simulink model "sampleModel51"  (R2021b)
settings: Solver=VariableStepAuto  StartTime=0.0  StopTime=10.0  RelTol=1e-3
undefined symbols (not defined in the file or in its folder): DiscIntNeverNeededParam, Newton, Raphson
libraries: simulink x10
settings Model: Creator=user  LastModifiedBy=user

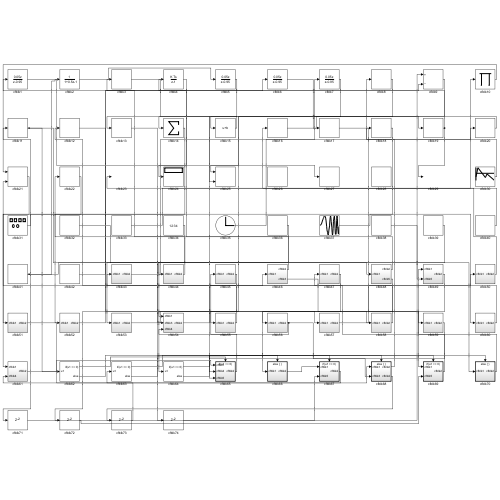
[thumbnail: Simulink's stored preview of the top-level diagram]
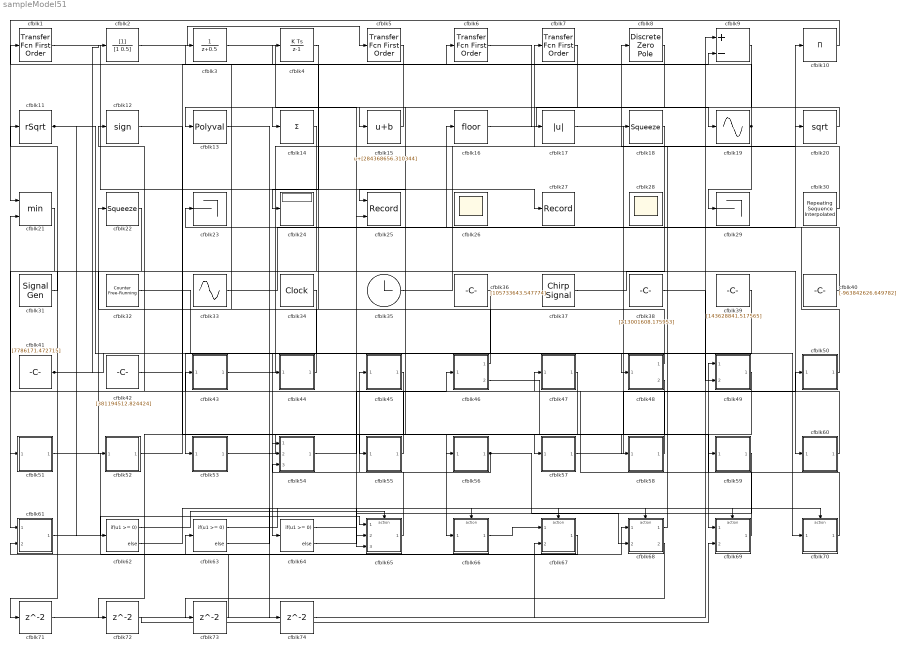
== system sampleModel51 ==
  cfblk{1,5..7} (4 alike) : simulink/Discrete/Transfer Fcn First Order  PoleZ=0.95  ICPrevOutput=0.0  DoSatur=off
  cfblk10 : Product  Inputs=*
  cfblk11 : Sqrt  Operator=rSqrt  AlgorithmType=Newton-Raphson  SaturateOnIntegerOverflow=on
  cfblk12 : Signum
  cfblk13 : Polyval  Coefs=[ +2.081618890e-019, -1.441693666e-014, +4.719686976e-010, -8.536869453e-006, +1.621573104e-001, -8.087801117e+001 ]
  cfblk14 : Sum  Inputs=+
  cfblk15 : Bias  Bias=[284368656.310344]
  cfblk16 : Rounding
  cfblk17 : Abs
  cfblk18 : Squeeze
  cfblk19 : Sin  TimeSource=Use external signal  SampleTime=0
  cfblk2 : DiscreteFilter  SampleTime=1
  cfblk20 : Sqrt  SaturateOnIntegerOverflow=on
  cfblk21 : MinMax  Inputs=2
  cfblk22 : Squeeze
  cfblk23 : Terminator
  cfblk24 : Display
  cfblk25 : Record  FileSettingsInternal="{\"entries\":[{\"content\":{\"excelSettings\":{\"content\":{},\"type\":\"Streamout.ExcelSettings\"}},\"type\":\"Streamout.FileSettingStorage\",\"uuid\":\"25a07257-a86f-477b-952e-0e759ef5e051\"}],\"packageUris\":[\"http://schema.mathworks.com/mf0/streamout_blocks/R2020a\"],\"version\":\"1.0\"}"  Layout=[1 1]  SignalsInternal="{\"entries\":[{\"content\":{\"signals\":[{\"content\":{\"blockPath\":[\"sampleModel51/cfblk25\"],\"channel\":[],\"dimensions\":[1],\"domain\":\"sampleModel51/cfblk25\",\"lineColor\":\"#a2142f\",\"plots\":[1],\"port\":1,\"sid\":[\"\"],\"signalID\":1857,\"signalName\":\"cfblk7\"},\"type\":\"RecordBlkView.Signal\",\"uuid\":\"bc7b99ac-22d1-4a7a-8eb9-f05fbf7987ad\"},{\"content\":{\"blockPath\":[\"sampleModel51/cfblk25\"],\"channel\":[],\"dimensions\":[1],\"domain\":\"sampleModel51/cfblk25\",\"lineColor\":\"#139fff\",\"plots\":[1],\"port\":2,\"sid\":[\"\"],\"signalID\":1861,\"signalName\":\"cfblk8\"},\"type\":\"RecordBlkView.Signal\",\"uuid\":\"eec4487d-860f-4009-9e4b-d7d68678033c\"}]},\"type\":\"RecordBlkView.InputSignals\",\"uuid\":\"330df4c9-4a7c-4ca9-881d-def7613869be\"}],\"packageUris\":[\"http://schema.mathworks.com/mf0/streamout_blocks/R2020a\"],\"version\":\"1.0\"}"  VisualizationBindings="{\"xyplotplugin\":{\"info\":[{\"series\":[{\"bindingParametersList\":[{\"parameter\":\"X-Axis\",\"signalID\":1857,\"signalName\":\"cfblk7\"},{\"parameter\":\"Y-Axis\",\"signalID\":1861,\"signalName\":\"cfblk8\"}],\"seriesID\":23151}],\"subplotID\":1}]}}"  CompatibilityTag=XY
  cfblk26 : Scope
      settings: Floating=on
  cfblk27 : Record  FileSettingsInternal="{\"entries\":[{\"content\":{\"excelSettings\":{\"content\":{},\"type\":\"Streamout.ExcelSettings\"}},\"type\":\"Streamout.FileSettingStorage\",\"uuid\":\"a12ccd90-a1d8-4ecd-8f26-21958fc88e0b\"}],\"packageUris\":[\"http://schema.mathworks.com/mf0/streamout_blocks/R2020a\"],\"version\":\"1.0\"}"  SignalsInternal="{\"entries\":[{\"content\":{\"signals\":[{\"content\":{\"blockPath\":[\"sampleModel51/cfblk27\"],\"channel\":[],\"dimensions\":[1],\"domain\":\"sampleModel51/cfblk27\",\"lineColor\":\"#b746ff\",\"plots\":[1],\"port\":1,\"sid\":[\"\"],\"signalID\":1853,\"signalName\":\"cfblk1\"},\"type\":\"RecordBlkView.Signal\",\"uuid\":\"1f1b1c54-a698-4fa8-9717-1515f275c3ed\"}]},\"type\":\"RecordBlkView.InputSignals\",\"uuid\":\"6aba2456-39ed-4904-9406-7c7f8254458a\"}],\"packageUris\":[\"http://schema.mathworks.com/mf0/streamout_blocks/R2020a\"],\"version\":\"1.0\"}"  VisualizationBindings="{\"sparklinesplugin\":{\"info\":[{\"bindingParametersList\":[],\"subplotID\":1}]}}"
  cfblk28 : Scope
      settings: Floating=on
  cfblk29 : Terminator
  cfblk3 : DiscreteTransferFcn  SampleTime=1
  cfblk30 : simulink/Sources/Repeating Sequence Interpolated  OutValues=[-278627430.459222, 439164858.532469, -328851896.173823, -43963004.255277, -552329955.086711]  TimeValues=[0 0.1 0.5 0.6 1].'  LookUpMeth=Use Input Nearest  tsamp=0.01  OutMin=[]  OutMax=[]  OutDataTypeStr=double  OutputDataTypeScalingMode=double  OutDataType=fixdt(0,8)  OutScaling=2^-10
  cfblk31 : SignalGenerator  Amplitude=[243590977.755836]  Units=rad/sec
  cfblk32 : simulink/Sources/Counter Free-Running  NumBits=[9.000000]  tsamp=-1
  cfblk33 : Sin  Amplitude=[-822452745.496460]  Bias=[355937665.423615]  SampleTime=0
  cfblk34 : DigitalClock
  cfblk35 : Clock
  cfblk36 : Constant  Value=[105733643.547774]  SampleTime=1
  cfblk37 : simulink/Sources/Chirp Signal  f1=[-199962809.726746]  T=[147891668.344843]  f2=[-456672976.291181]
  cfblk38 : Constant  Value=[213001608.175953]  SampleTime=1
  cfblk39 : Constant  Value=[143628841.517565]  SampleTime=1
  cfblk4 : DiscreteIntegrator  ICPrevOutput=DiscIntNeverNeededParam  ICPrevScaledInput=DiscIntNeverNeededParam
  cfblk40 : Constant  Value=[-963842626.649782]  SampleTime=1
  cfblk41 : Constant  Value=[7786171.472715]  SampleTime=1
  cfblk42 : Constant  Value=[381194512.824424]  SampleTime=1
  cfblk43 : Subsystem
  cfblk44 : Subsystem
  cfblk45 : Subsystem
  cfblk46 : Subsystem
  cfblk47 : Subsystem
  cfblk48 : Subsystem
  cfblk49 : Subsystem
  cfblk50 : Subsystem
  cfblk51 : Subsystem
  cfblk52 : Subsystem
  cfblk53 : Subsystem
  cfblk54 : Subsystem
  cfblk55 : Subsystem
  cfblk56 : Subsystem
  cfblk57 : Subsystem
  cfblk58 : Subsystem
  cfblk59 : Subsystem
  cfblk60 : Subsystem
  cfblk61 : Subsystem
  cfblk62 : If  IfExpression=u1 >= 0  SampleTime=1
  cfblk63 : If  IfExpression=u1 >= 0  SampleTime=1
  cfblk64 : If  IfExpression=u1 >= 0  SampleTime=1
  cfblk65 : Subsystem  TreatAsAtomicUnit=on
  cfblk66 : Subsystem  TreatAsAtomicUnit=on
  cfblk67 : Subsystem  TreatAsAtomicUnit=on
  cfblk68 : Subsystem  TreatAsAtomicUnit=on
  cfblk69 : Subsystem  TreatAsAtomicUnit=on
  cfblk70 : Subsystem  TreatAsAtomicUnit=on
  cfblk{71..74} (4 alike) : Delay  SampleTime=1
  cfblk8 : DiscreteZeroPole  Poles=[0 0.5]  Gain=1
  cfblk9 : Sum  Inputs=+-
  wires:
  cfblk65/1(cfblk2) -> cfblk45/1(cfblk1)
  cfblk39/1 -> cfblk53/1(cfblk1)
  cfblk2/1 -> cfblk5/1
  cfblk51/1(cfblk2) -> cfblk68/1(cfblk1)
  cfblk61/1(cfblk2) -> cfblk65/1(cfblk1)
  cfblk37/1 -> cfblk60/1(cfblk1)
  cfblk16/1 -> cfblk19/1
  cfblk1/1 -> cfblk27/1
  cfblk50/1(cfblk2) -> cfblk23/1
  cfblk44/1(cfblk2) -> cfblk22/1
  cfblk69/1(cfblk2) -> cfblk49/1(cfblk1)
  cfblk5/1 -> cfblk14/1
  cfblk59/1(cfblk2) -> cfblk65/2(cfblk4)
  cfblk10/1 -> cfblk21/1
  cfblk57/1(cfblk2) -> cfblk50/1(cfblk1)
  cfblk41/1 -> cfblk2/1, cfblk48/1(cfblk1)
  cfblk15/1 -> cfblk13/1
  cfblk12/1 -> cfblk58/1(cfblk1)
  cfblk35/1 -> cfblk7/1
  cfblk31/1 -> cfblk11/1
  cfblk60/1(cfblk2) -> cfblk12/1
  cfblk40/1 -> cfblk16/1
  cfblk33/1 -> cfblk10/1
  cfblk36/1 -> cfblk64/1
  cfblk47/1(cfblk2) -> cfblk66/1(cfblk1)
  cfblk38/1 -> cfblk49/2(cfblk5)
  cfblk55/1(cfblk2) -> cfblk43/1(cfblk1)
  cfblk9/1 -> cfblk55/1(cfblk1)
  cfblk32/1 -> cfblk70/1(cfblk1)
  cfblk54/1(cfblk2) -> cfblk46/1(cfblk1)
  cfblk49/1(cfblk2) -> cfblk56/1(cfblk1)
  cfblk20/1 -> cfblk15/1
  cfblk58/1(cfblk2) -> cfblk21/2
  cfblk17/1 -> cfblk69/1(cfblk1)
  cfblk30/1 -> cfblk8/1
  cfblk52/1(cfblk2) -> cfblk6/1
  cfblk22/1 -> cfblk61/1(cfblk1)
  cfblk53/1(cfblk2) -> cfblk57/1(cfblk1)
  cfblk6/1 -> cfblk17/1
  cfblk70/1(cfblk2) -> cfblk47/1(cfblk1)
  cfblk3/1 -> cfblk65/3(cfblk5)
  cfblk66/1(cfblk2) -> cfblk67/1(cfblk1)
  cfblk68/1(cfblk2) -> cfblk18/1
  cfblk43/1(cfblk2) -> cfblk20/1
  cfblk21/1 -> cfblk51/1(cfblk1)
  cfblk4/1 -> cfblk24/1
  cfblk46/1(cfblk2) -> cfblk4/1
  cfblk67/1(cfblk2) -> cfblk61/2(cfblk4)
  cfblk7/1 -> cfblk25/1
  cfblk14/1 -> cfblk52/1(cfblk1)
  cfblk42/1 -> cfblk9/2
  cfblk8/1 -> cfblk25/2
  cfblk56/1(cfblk2) -> cfblk68/2(cfblk3), cfblk54/3(cfblk4)
  cfblk11/1 -> cfblk44/1(cfblk1), cfblk62/1
  cfblk46/2(cfblk3) -> cfblk59/1(cfblk1)
  cfblk19/1 -> cfblk29/1, cfblk1/1
  cfblk48/1(cfblk2) -> cfblk3/1
  cfblk48/2(cfblk5) -> cfblk54/1(cfblk1)
  cfblk34/1 -> cfblk54/2(cfblk3)
  cfblk62/1 -> cfblk65/Action
  cfblk62/2 -> cfblk66/Action
  cfblk63/1 -> cfblk67/Action
  cfblk63/2 -> cfblk68/Action
  cfblk64/1 -> cfblk69/Action
  cfblk64/2 -> cfblk70/Action
  cfblk18/1 -> cfblk71/1
  cfblk71/1 -> cfblk67/2(cfblk5)
  cfblk45/1(cfblk2) -> cfblk72/1
  cfblk72/1 -> cfblk69/2(cfblk5)
  cfblk68/2(cfblk4) -> cfblk73/1
  cfblk73/1 -> cfblk63/1
  cfblk13/1 -> cfblk74/1
  cfblk74/1 -> cfblk9/1

== system sampleModel51/cfblk43 ==
  cfblk1 : Inport
  cfblk3 : Product  Inputs=*
  cfblk2 : Outport
  wires:
  cfblk1/1 -> cfblk2/1, cfblk3/1

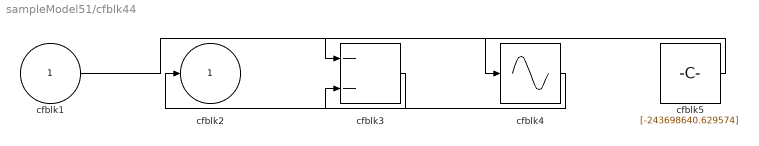
== system sampleModel51/cfblk44 ==
  cfblk1 : Inport
  cfblk3 : Sum  Inputs=--
  cfblk4 : Sin  TimeSource=Use external signal  SampleTime=0
  cfblk5 : Constant  Value=[-243698640.629574]  SampleTime=1
  cfblk2 : Outport
  wires:
  cfblk5/1 -> cfblk3/1
  cfblk3/1 -> cfblk2/1
  cfblk4/1 -> cfblk3/2
  cfblk1/1 -> cfblk4/1

== system sampleModel51/cfblk45 ==
  cfblk1 : Inport
  cfblk3 : Bias  Bias=[345475701.339548]
  cfblk2 : Outport
  wires:
  cfblk1/1 -> cfblk3/1
  cfblk3/1 -> cfblk2/1

== system sampleModel51/cfblk46 ==
  cfblk1 : Inport
  cfblk2 : Outport
  cfblk3 : Outport  Port=2
  wires:
  cfblk1/1 -> cfblk3/1, cfblk2/1

== system sampleModel51/cfblk47 ==
  cfblk1 : Inport
  cfblk3 : Sqrt  SaturateOnIntegerOverflow=on
  cfblk2 : Outport
  wires:
  cfblk1/1 -> cfblk3/1
  cfblk3/1 -> cfblk2/1

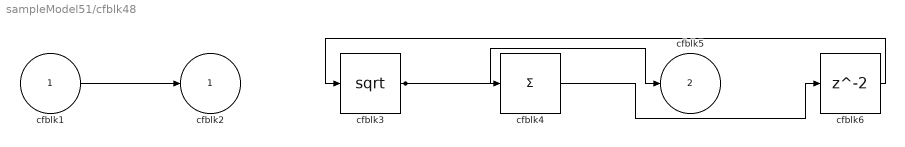
== system sampleModel51/cfblk48 ==
  cfblk1 : Inport
  cfblk3 : Sqrt  SaturateOnIntegerOverflow=on
  cfblk4 : Sum  Inputs=+
  cfblk6 : Delay  SampleTime=1
  cfblk2 : Outport
  cfblk5 : Outport  Port=2
  wires:
  cfblk3/1 -> cfblk5/1, cfblk4/1
  cfblk1/1 -> cfblk2/1
  cfblk4/1 -> cfblk6/1
  cfblk6/1 -> cfblk3/1

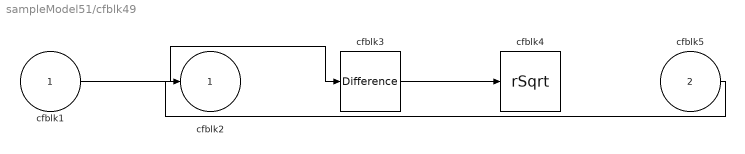
== system sampleModel51/cfblk49 ==
  cfblk1 : Inport
  cfblk5 : Inport  Port=2
  cfblk3 : simulink/Discrete/Difference  ICPrevInput=0.0  OutMin=[]  OutMax=[]  OutDataTypeStr=Inherit: Inherit via back propagation  OutDataType=fixdt(1, 16)  OutScaling=2^-10  DoSatur=off
  cfblk4 : Sqrt  Operator=rSqrt  AlgorithmType=Newton-Raphson  SaturateOnIntegerOverflow=on
  cfblk2 : Outport
  wires:
  cfblk3/1 -> cfblk4/1
  cfblk1/1 -> cfblk3/1
  cfblk5/1 -> cfblk2/1

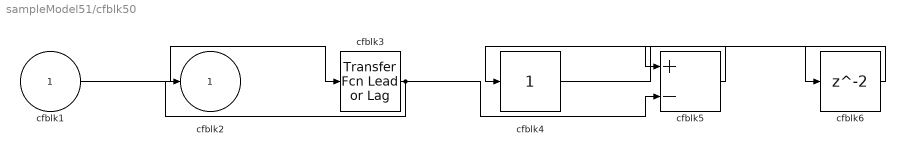
== system sampleModel51/cfblk50 ==
  cfblk1 : Inport
  cfblk3 : simulink/Discrete/Transfer Fcn Lead or Lag  PoleZ=0.95  ZeroZ=0.75  ICPrevOutput=0.0  ICPrevInput=0.0  DoSatur=off
      settings: SourceProductBaseCode=SL
  cfblk4 : simulink/Math Operations/Slider Gain  gain=1  low=0  high=2
  cfblk5 : Sum  Inputs=+-
  cfblk6 : Delay  SampleTime=1
  cfblk2 : Outport
  wires:
  cfblk1/1 -> cfblk3/1
  cfblk3/1 -> cfblk2/1, cfblk5/2
  cfblk5/1 -> cfblk4/1
  cfblk4/1 -> cfblk6/1
  cfblk6/1 -> cfblk5/1

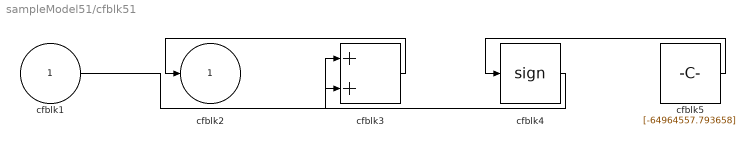
== system sampleModel51/cfblk51 ==
  cfblk1 : Inport
  cfblk3 : Sum
  cfblk4 : Signum
  cfblk5 : Constant  Value=[-64964557.793658]  SampleTime=1
  cfblk2 : Outport
  wires:
  cfblk5/1 -> cfblk4/1
  cfblk3/1 -> cfblk2/1
  cfblk4/1 -> cfblk3/1
  cfblk1/1 -> cfblk3/2

== system sampleModel51/cfblk52 ==
  cfblk1 : Inport
  cfblk3 : Rounding
  cfblk2 : Outport
  wires:
  cfblk1/1 -> cfblk3/1
  cfblk3/1 -> cfblk2/1

== system sampleModel51/cfblk53 ==
  cfblk1 : Inport
  cfblk3 : Sum  Inputs=--
  cfblk2 : Outport
  wires:
  cfblk1/1 -> cfblk2/1, cfblk3/1, cfblk3/2

== system sampleModel51/cfblk54 ==
  cfblk1 : Inport
  cfblk3 : Inport  Port=2
  cfblk4 : Inport  Port=3
  cfblk2 : Outport
  wires:
  cfblk3/1 -> cfblk2/1

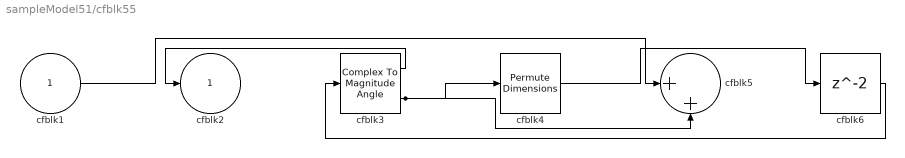
== system sampleModel51/cfblk55 ==
  cfblk1 : Inport
  cfblk3 : ComplexToMagnitudeAngle
  cfblk4 : PermuteDimensions
  cfblk5 : Sum  Inputs=|++
  cfblk6 : Delay  SampleTime=1
  cfblk2 : Outport
  wires:
  cfblk3/1 -> cfblk2/1
  cfblk1/1 -> cfblk5/1
  cfblk3/2 -> cfblk4/1, cfblk5/2
  cfblk4/1 -> cfblk6/1
  cfblk6/1 -> cfblk3/1

== system sampleModel51/cfblk56 ==
  cfblk1 : Inport
  cfblk3 : Bias  Bias=[-496468603.087499]
  cfblk4 : Constant  Value=[178339458.537711]  SampleTime=1
  cfblk2 : Outport
  wires:
  cfblk1/1 -> cfblk3/1
  cfblk3/1 -> cfblk2/1

== system sampleModel51/cfblk57 ==
  cfblk1 : Inport
  cfblk3 : Delay  DelayLengthSource=Input port  SampleTime=1
      settings: InputPortMap=u0,p1
  cfblk4 : Constant  Value=[-820685730.446150]  SampleTime=1
  cfblk2 : Outport
  wires:
  cfblk1/1 -> cfblk3/1
  cfblk4/1 -> cfblk3/2
  cfblk3/1 -> cfblk2/1

== system sampleModel51/cfblk58 ==
  cfblk1 : Inport
  cfblk3 : Constant  Value=[-362818715.919732]  SampleTime=1
  cfblk2 : Outport
  wires:
  cfblk3/1 -> cfblk2/1

== system sampleModel51/cfblk59 ==
  cfblk1 : Inport
  cfblk3 : Sqrt  SaturateOnIntegerOverflow=on
  cfblk2 : Outport
  wires:
  cfblk3/1 -> cfblk2/1
  cfblk1/1 -> cfblk3/1

== system sampleModel51/cfblk60 ==
  cfblk1 : Inport
  cfblk3 : ComplexToRealImag
  cfblk2 : Outport
  wires:
  cfblk1/1 -> cfblk3/1
  cfblk3/1 -> cfblk2/1

== system sampleModel51/cfblk61 ==
  cfblk1 : Inport
  cfblk4 : Inport  Port=2
  cfblk3 : Assignment  DiagnosticForDimensions=Warning  IndexOptions=Index vector (dialog)  Indices=1  OutputSizes=1
  cfblk2 : Outport
  wires:
  cfblk3/1 -> cfblk2/1
  cfblk4/1 -> cfblk3/1
  cfblk1/1 -> cfblk3/2

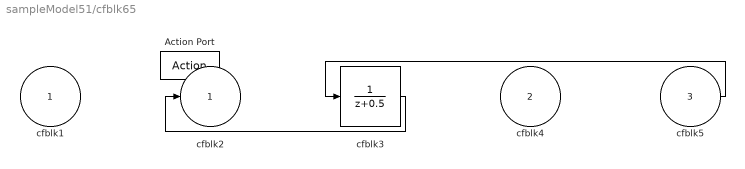
== system sampleModel51/cfblk65 ==
  cfblk1 : Inport
  cfblk4 : Inport  Port=2
  cfblk5 : Inport  Port=3
  Action Port : ActionPort  ActionPortLabel=if(u1 >= 0)
  cfblk3 : DiscreteTransferFcn
  cfblk2 : Outport
  wires:
  cfblk5/1 -> cfblk3/1
  cfblk3/1 -> cfblk2/1

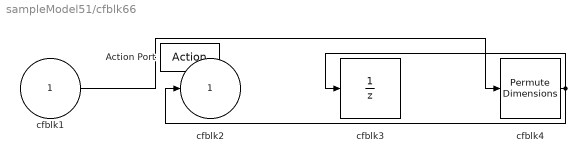
== system sampleModel51/cfblk66 ==
  cfblk1 : Inport
  Action Port : ActionPort  ActionPortLabel=else
  cfblk3 : UnitDelay  SampleTime=-1  HasFrameUpgradeWarning=on
  cfblk4 : PermuteDimensions
  cfblk2 : Outport
  wires:
  cfblk4/1 -> cfblk2/1, cfblk3/1
  cfblk1/1 -> cfblk4/1

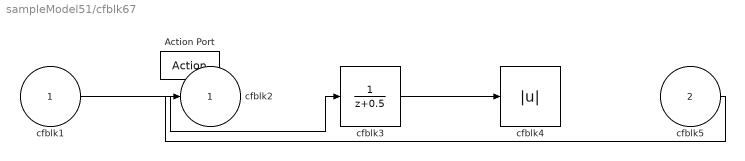
== system sampleModel51/cfblk67 ==
  cfblk1 : Inport
  cfblk5 : Inport  Port=2
  Action Port : ActionPort  ActionPortLabel=if(u1 >= 0)
  cfblk3 : DiscreteTransferFcn
  cfblk4 : Abs
  cfblk2 : Outport
  wires:
  cfblk1/1 -> cfblk3/1
  cfblk5/1 -> cfblk2/1
  cfblk3/1 -> cfblk4/1

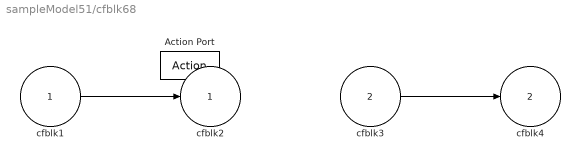
== system sampleModel51/cfblk68 ==
  cfblk1 : Inport
  cfblk3 : Inport  Port=2
  Action Port : ActionPort  ActionPortLabel=else
  cfblk2 : Outport
  cfblk4 : Outport  Port=2
  wires:
  cfblk3/1 -> cfblk4/1
  cfblk1/1 -> cfblk2/1

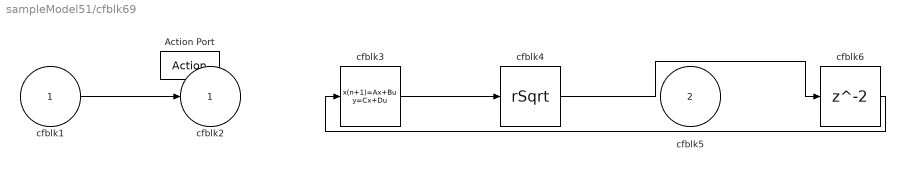
== system sampleModel51/cfblk69 ==
  cfblk1 : Inport
  cfblk5 : Inport  Port=2
  Action Port : ActionPort  ActionPortLabel=if(u1 >= 0)
  cfblk3 : DiscreteStateSpace  SampleTime=-1
  cfblk4 : Sqrt  Operator=rSqrt  AlgorithmType=Newton-Raphson  SaturateOnIntegerOverflow=on
  cfblk6 : Delay
  cfblk2 : Outport
  wires:
  cfblk3/1 -> cfblk4/1
  cfblk1/1 -> cfblk2/1
  cfblk4/1 -> cfblk6/1
  cfblk6/1 -> cfblk3/1

== system sampleModel51/cfblk70 ==
  cfblk1 : Inport
  Action Port : ActionPort  ActionPortLabel=else
  cfblk3 : Signum
  cfblk2 : Outport
  wires:
  cfblk1/1 -> cfblk3/1
  cfblk3/1 -> cfblk2/1
